simulink model "Dynamics_RotationalEoM_TH"  (Simulink 7.8)
settings: Solver=ode45  StartTime=0.0  StopTime=10  RelTol=1e-3
libraries: AeroSim x3
settings Model: Creator=Ryan  LastModifiedBy=Ryan

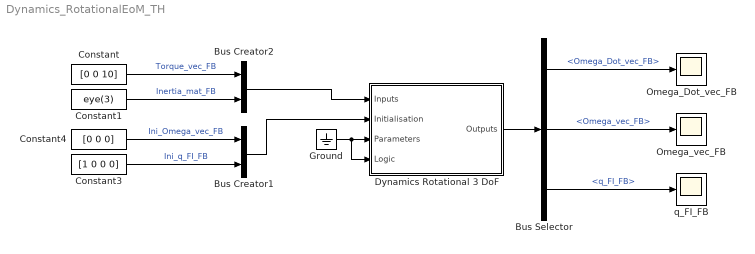
== system Dynamics_RotationalEoM_TH ==
  Bus Creator1 : BusCreator  Inputs=2
  Bus Creator2 : BusCreator  Inputs=2
  Bus Selector : BusSelector  OutputSignals=Omega_Dot_vec_FB,Omega_vec_FB,q_FI_FB
  Constant : Constant  Value=[0 0 10]
  Constant1 : Constant  Value=eye(3)
  Constant3 : Constant  Value=[1 0 0 0]
  Constant4 : Constant  Value=[0 0 0]
  Dynamics Rotational 3 DoF : Subsystem
  Ground : Ground
  Omega_Dot_vec_FB : Scope
  Omega_vec_FB : Scope
  q_FI_FB : Scope
      settings: SaveName=ScopeData2
  wires:
  Ground/1 -> Dynamics Rotational 3 DoF/3(Parameters), Dynamics Rotational 3 DoF/4(Logic)
  Constant/1 -> Bus Creator2/1  "Torque_vec_FB"
  Bus Creator2/1 -> Dynamics Rotational 3 DoF/1(Inputs)
  Bus Creator1/1 -> Dynamics Rotational 3 DoF/2(Initialisation)
  Dynamics Rotational 3 DoF/1(Outputs) -> Bus Selector/1
  Bus Selector/1 -> Omega_Dot_vec_FB/1  "<Omega_Dot_vec_FB>"
  Bus Selector/2 -> Omega_vec_FB/1  "<Omega_vec_FB>"
  Bus Selector/3 -> q_FI_FB/1  "<q_FI_FB>"
  Constant4/1 -> Bus Creator1/1  "Ini_Omega_vec_FB"
  Constant3/1 -> Bus Creator1/2  "Ini_q_FI_FB"
  Constant1/1 -> Bus Creator2/2  "Inertia_mat_FB"

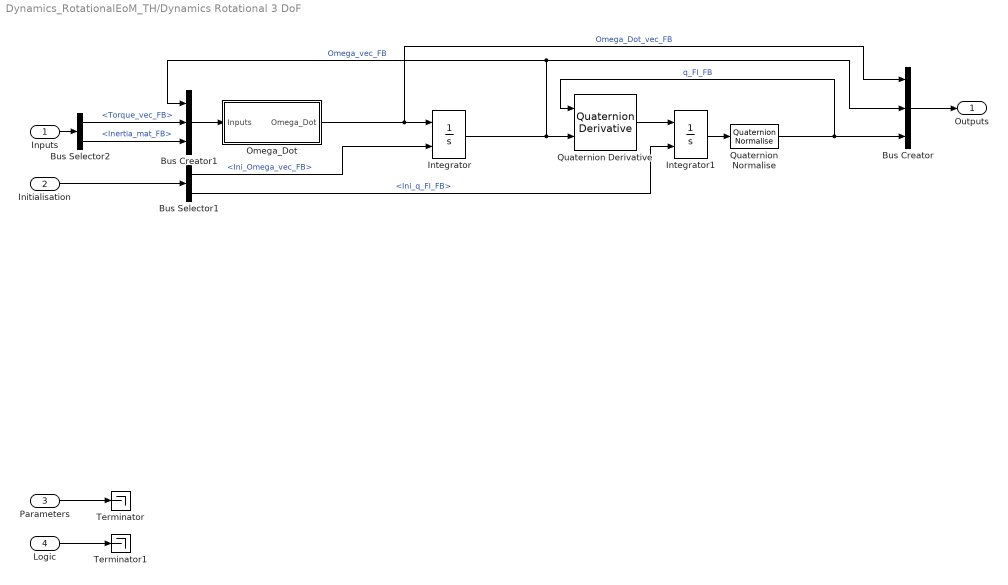
== system Dynamics_RotationalEoM_TH/Dynamics Rotational 3 DoF ==
  Inputs : Inport  OutDataTypeStr=Bus: Dynamics_RotationalEoM_Inputs
  Initialisation : Inport  Port=2  OutDataTypeStr=Bus: Dynamics_RotationalEoM_Initialisation
  Parameters : Inport  Port=3
  Logic : Inport  Port=4
  Bus Creator : BusCreator  Inputs=3
  Bus Creator1 : BusCreator  Inputs=3
  Bus Selector1 : BusSelector  OutputSignals=Ini_Omega_vec_FB,Ini_q_FI_FB
  Bus Selector2 : BusSelector  OutputSignals=Torque_vec_FB,Inertia_mat_FB
  Integrator : Integrator  InitialConditionSource=external
  Integrator1 : Integrator  InitialConditionSource=external
  Omega_Dot : Subsystem
  Quaternion Derivative : AeroSim/Mathematics/Quaternion Derivative
  Quaternion Normalise : AeroSim/Mathematics/Quaternion Normalise
  Terminator : Terminator
  Terminator1 : Terminator
  Outputs : Outport  OutDataTypeStr=Bus: Dynamics_RotationalEoM_Outputs
  wires:
  Parameters/1 -> Terminator/1
  Logic/1 -> Terminator1/1
  Initialisation/1 -> Bus Selector1/1
  Bus Creator/1 -> Outputs/1
  Omega_Dot/1(Omega_Dot) -> Integrator/1, Bus Creator/1  "Omega_Dot_vec_FB"
  Bus Selector1/1 -> Integrator/2  "<Ini_Omega_vec_FB>"
  Integrator/1 -> Quaternion Derivative/2, Bus Creator/2, Bus Creator1/1  "Omega_vec_FB"
  Quaternion Derivative/1 -> Integrator1/1
  Bus Selector1/2 -> Integrator1/2  "<Ini_q_FI_FB>"
  Integrator1/1 -> Quaternion Normalise/1
  Quaternion Normalise/1 -> Quaternion Derivative/1, Bus Creator/3  "q_FI_FB"
  Inputs/1 -> Bus Selector2/1
  Bus Selector2/2 -> Bus Creator1/3  "<Inertia_mat_FB>"
  Bus Selector2/1 -> Bus Creator1/2  "<Torque_vec_FB>"
  Bus Creator1/1 -> Omega_Dot/1(Inputs)

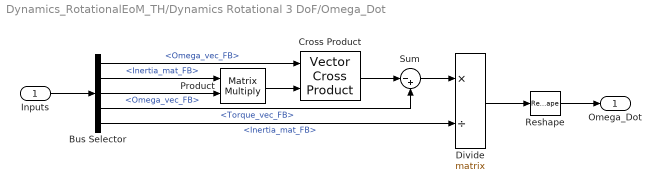
== system Dynamics_RotationalEoM_TH/Dynamics Rotational 3 DoF/Omega_Dot ==
  Inputs : Inport
  Bus Selector : BusSelector  OutputSignals=Omega_vec_FB,Inertia_mat_FB,Omega_vec_FB,Torque_vec_FB,Inertia_mat_FB
  Cross Product : AeroSim/Mathematics/Vector Cross Product
  Divide : Product  Inputs=*/  Multiplication=Matrix(*)
  Product : Product  Multiplication=Matrix(*)  RndMeth=Zero
  Reshape : Reshape
  Sum : Sum  Inputs=|-+
  Omega_Dot : Outport
  wires:
  Inputs/1 -> Bus Selector/1
  Product/1 -> Cross Product/2
  Cross Product/1 -> Sum/1
  Bus Selector/1 -> Cross Product/1  "<Omega_vec_FB>"
  Bus Selector/3 -> Product/2  "<Omega_vec_FB>"
  Bus Selector/4 -> Sum/2  "<Torque_vec_FB>"
  Sum/1 -> Divide/1
  Divide/1 -> Reshape/1
  Bus Selector/2 -> Product/1  "<Inertia_mat_FB>"
  Bus Selector/5 -> Divide/2  "<Inertia_mat_FB>"
  Reshape/1 -> Omega_Dot/1
